simulink model "mapp_4_fir_4_str"  (R2018b)
settings: Solver=ode45  StartTime=0.0  StopTime=200  RelTol=1e-3  EnableMultiTasking=on
undefined symbols (not defined in the file or in its folder): CMD_ci_Re_0, CMD_ci_Re_21, CMD_ci_str_0, CMD_ci_str_1, CMD_ci_str_10, CMD_ci_str_11, CMD_ci_str_12, CMD_ci_str_13, CMD_ci_str_14, CMD_ci_str_15, CMD_ci_str_16, CMD_ci_str_17, CMD_ci_str_18, CMD_ci_str_19, CMD_ci_str_2, CMD_ci_str_20, CMD_ci_str_21, CMD_ci_str_3, CMD_ci_str_4, CMD_ci_str_5, CMD_ci_str_6, CMD_ci_str_7, CMD_ci_str_8, CMD_ci_str_9, CMD_decr_0, CMD_deka_down, CMD_deka_up, CMD_fb, CMD_FB_mult, CMD_Firprg_0, CMD_Firprg_1, CMD_gain, CMD_ind_mult, CMD_ind_mult_1, CMD_ind_mult_2, CMD_ind_mult_3, CMD_ind_mult_4, CMD_ind_stuk, CMD_ind_vol, CMD_ind_vol_1, CMD_ind_vol_2, CMD_ind_vol_3, CMD_ind_vol_4, CMD_init_dac, CMD_init_sw, CMD_molot_string, CMD_nl, CMD_nl_sl, CMD_omega_0, CMD_out_vol, CMD_param_0, CMD_param_5, CMD_pedal, CMD_reset, CMD_rst, CMD_shape_0, CMD_step_down, CMD_step_up, CMD_str_svertk, ind_mult_0 ... (+10)
libraries: xbsIndex_r4 x3300
(part 3 of 16)

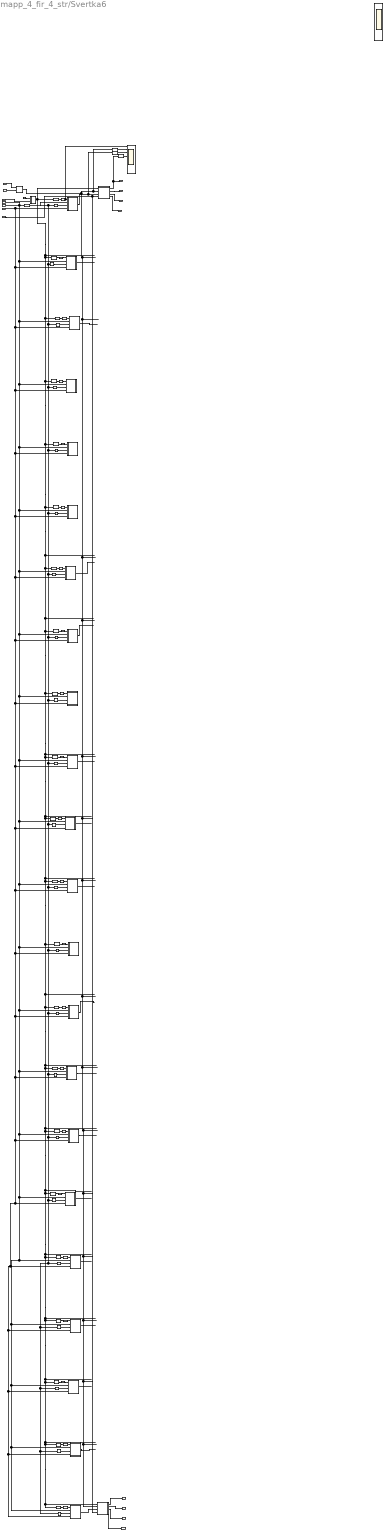
== system mapp_4_fir_4_str/Svertka6 ==
  A_sunn[j] : Inport
  m_dat : Inport  Port=2
  m_addr : Inport  Port=3
  m_en : Inport  Port=4
  start : Inport  Port=5
  FB : Inport  Port=6
  reset : Inport  Port=7
  Constant17 : xbsIndex_r4/Constant  const=531  gui_display_data_type=Fixed-point  arith_type=Unsigned  n_bits=12  bin_pt=0  preci_type=Single  exp_width=8  frac_width=24  explicit_period=off  period=1  equ=P=C  opselect=C  inp2=PCIN>>17  opr=+  inp1=P  carry=CIN  dbl_ovrd=off  block_type=constant
      settings: block_version=VER_STRING_GOES_HERE
  Convert1 : xbsIndex_r4/Convert  gui_display_data_type=Floating-point  arith_type=Floating-point  n_bits=48  bin_pt=0  float_type=Single  exp_bits=8  fraction_bits=24  quantization="Round  (unbiased: +/- Inf)"  overflow=Saturate  en=off  latency=0  pipeline=off  dbl_ovrd=off  block_type=convert
  Convert12 : xbsIndex_r4/Convert  gui_display_data_type=Floating-point  arith_type=Floating-point  n_bits=48  bin_pt=0  float_type=Single  exp_bits=8  fraction_bits=24  quantization="Round  (unbiased: +/- Inf)"  overflow=Saturate  en=off  latency=0  pipeline=off  dbl_ovrd=off  block_type=convert
  Convert2 : xbsIndex_r4/Convert  gui_display_data_type=Floating-point  arith_type=Floating-point  n_bits=48  bin_pt=0  float_type=Single  exp_bits=8  fraction_bits=24  quantization="Round  (unbiased: +/- Inf)"  overflow=Saturate  en=off  latency=0  pipeline=off  dbl_ovrd=off  block_type=convert
  Count : Subsystem
  Delay{1..9,12..16,18..24,278} (22 alike) : xbsIndex_r4/Delay  rst=off  infoeditControl=Selection of Reset will increase slice count due to use of real FFs and instead of SRLs  en=off  latency=127  reg_retiming=off  dbl_ovrd=off  block_type=delay
  Delay{10..11,28,44,58,72,85,100,114,128,141,155,169,182,197,211,225,238,253,267,295,308} (22 alike) : xbsIndex_r4/Delay  rst=off  infoeditControl=Selection of Reset will increase slice count due to use of real FFs and instead of SRLs  en=off  latency=1  reg_retiming=on  dbl_ovrd=off  block_type=delay
      settings: xl_area=[16 32 0 0 0 0 0]  block_version=VER_STRING_GOES_HERE
  Delay{17,27,33,49,63,77,90,105,119,133,146,160,174,187,202,216,230,243,258,272,300,313} (22 alike) : xbsIndex_r4/Delay  rst=off  infoeditControl=Selection of Reset will increase slice count due to use of real FFs and instead of SRLs  en=off  latency=1  reg_retiming=off  dbl_ovrd=off  block_type=delay
  Mult22 : xbsIndex_r4/Mult  precision=Full  arith_type="Signed  (2's comp)"  n_bits=16  bin_pt=14  quantization=Truncate  overflow=Wrap  en=off  latency=6  use_behavioral_HDL=on  opt=Speed  use_embedded=on  optimum_pipeline=off  pipeline=on  dbl_ovrd=off  use_rpm=on  placement_style=Triangular  block_type=mult
  RSlice1 : xbsIndex_r4/Slice  nbits=10  boolean_output=off  mode=Lower Bit Location + Width  bit1=0  base1=MSB of Input  bit0=0  base0=LSB of Input  dbl_ovrd=off  block_type=slice
      settings: block_version=VER_STRING_GOES_HERE
  Scope1 : Scope  NumInputPorts=8
  Scope3 : Scope  NumInputPorts=9
  accum_0 : Subsystem
  accum_1 : Subsystem
  ci_re_0 : Subsystem
  ci_re_1 : Subsystem
  ci_re_10 : Subsystem
  ci_re_11 : Subsystem
  ci_re_12 : Subsystem
  ci_re_13 : Subsystem
  ci_re_14 : Subsystem
  ci_re_15 : Subsystem
  ci_re_16 : Subsystem
  ci_re_17 : Subsystem
  ci_re_18 : Subsystem
  ci_re_19 : Subsystem
  ci_re_2 : Subsystem
  ci_re_20 : Subsystem
  ci_re_21 : Subsystem
  ci_re_3 : Subsystem
  ci_re_4 : Subsystem
  ci_re_5 : Subsystem
  ci_re_6 : Subsystem
  ci_re_7 : Subsystem
  ci_re_8 : Subsystem
  ci_re_9 : Subsystem
  nota_0 : Outport
  nota_87 : Outport  Port=2
  nota_1 : Outport  Port=3
  nota_86 : Outport  Port=4
  nota_2 : Outport  Port=5
  nota_85 : Outport  Port=6
  nota_3 : Outport  Port=7
  nota_84 : Outport  Port=8
  wires:
  start/1 -> Count/2(start)
  Delay27/1 -> Scope3/1, ci_re_0/1(addr)
  m_en/1 -> ci_re_0/4(m_en), ci_re_1/4(m_en), ci_re_6/4(m_en), ci_re_7/4(m_en), ci_re_9/4(m_en), ci_re_10/4(m_en), ci_re_11/4(m_en), ci_re_12/4(m_en), ci_re_13/4(m_en), ci_re_14/4(m_en), ci_re_15/4(m_en), ci_re_16/4(m_en), ci_re_18/4(m_en), ci_re_19/4(m_en), ci_re_20/4(m_en), ci_re_21/4(m_en), ci_re_17/4(m_en), ci_re_8/4(m_en), ci_re_5/4(m_en), ci_re_4/4(m_en), ci_re_3/4(m_en), ci_re_2/4(m_en)
  Delay7/1 -> Delay27/1
  Constant17/1 -> Count/1(In1)
  m_addr/1 -> RSlice1/1
  Delay24/1 -> Delay17/1
  Delay17/1 -> ci_re_1/1(addr)
  Delay33/1 -> ci_re_2/1(addr)
  Delay23/1 -> Delay33/1
  Delay28/1 -> ci_re_2/3(m_addr)
  Delay44/1 -> ci_re_3/3(m_addr)
  Delay22/1 -> Delay49/1
  Delay49/1 -> ci_re_3/1(addr)
  Delay63/1 -> ci_re_4/1(addr)
  Delay21/1 -> Delay63/1
  Delay58/1 -> ci_re_4/3(m_addr)
  Delay77/1 -> ci_re_5/1(addr)
  Delay20/1 -> Delay77/1
  Delay72/1 -> ci_re_5/3(m_addr)
  Delay128/1 -> ci_re_9/3(m_addr)
  Delay15/1 -> Delay133/1
  Delay133/1 -> ci_re_9/1(addr)
  Delay114/1 -> ci_re_8/3(m_addr)
  Delay16/1 -> Delay119/1
  Delay119/1 -> ci_re_8/1(addr)
  Delay105/1 -> ci_re_7/1(addr)
  Delay18/1 -> Delay105/1
  Delay100/1 -> ci_re_7/3(m_addr)
  Delay85/1 -> ci_re_6/3(m_addr)
  Delay19/1 -> Delay90/1
  Delay90/1 -> ci_re_6/1(addr)
  Delay243/1 -> ci_re_14/1(addr)
  Delay238/1 -> ci_re_14/3(m_addr)
  Delay141/1 -> ci_re_15/3(m_addr)
  Delay146/1 -> ci_re_15/1(addr)
  Delay6/1 -> Delay146/1
  Delay160/1 -> ci_re_16/1(addr)
  Delay155/1 -> ci_re_16/3(m_addr)
  Delay5/1 -> Delay160/1
  Delay211/1 -> ci_re_12/3(m_addr)
  Delay216/1 -> ci_re_12/1(addr)
  Delay12/1 -> Delay216/1
  Delay174/1 -> ci_re_17/1(addr)
  Delay169/1 -> ci_re_17/3(m_addr)
  Delay4/1 -> Delay174/1
  Delay202/1 -> ci_re_11/1(addr)
  Delay13/1 -> Delay202/1
  Delay197/1 -> ci_re_11/3(m_addr)
  Delay8/1 -> Delay243/1
  Delay14/1 -> Delay187/1
  Delay187/1 -> ci_re_10/1(addr)
  Delay182/1 -> ci_re_10/3(m_addr)
  Delay230/1 -> ci_re_13/1(addr)
  Delay9/1 -> Delay230/1
  Delay225/1 -> ci_re_13/3(m_addr)
  Delay278/1 -> Delay272/1
  Delay272/1 -> ci_re_21/1(addr)
  RSlice1/1 -> Delay10/1, Delay11/1, Delay28/1, Delay44/1, Delay58/1, Delay72/1, Delay85/1, Delay100/1, Delay114/1, Delay128/1, Delay182/1, Delay238/1, Delay141/1, Delay155/1, Delay295/1, Delay308/1, Delay253/1, Delay267/1, Delay169/1, Delay225/1, Delay211/1, Delay197/1
  Delay258/1 -> ci_re_20/1(addr)
  Delay253/1 -> ci_re_20/3(m_addr)
  Delay313/1 -> ci_re_19/1(addr)
  Delay1/1 -> Delay258/1
  Delay295/1 -> ci_re_18/3(m_addr)
  Delay3/1 -> Delay300/1
  Delay300/1 -> ci_re_18/1(addr)
  Count/1(Out1) -> Delay24/1, Delay23/1, Delay22/1, Delay21/1, Delay20/1, Delay19/1, Delay18/1, Delay16/1, Delay15/1, Delay14/1, Delay13/1, Delay12/1, Delay9/1, Delay8/1, Delay6/1, Delay5/1, Delay4/1, Delay3/1, Delay2/1, Delay1/1, Delay278/1, accum_1/1(In1), accum_0/1(In1), Delay7/1
  Delay308/1 -> ci_re_19/3(m_addr)
  Delay2/1 -> Delay313/1
  m_dat/1 -> ci_re_1/2(m_data), ci_re_2/2(m_data), ci_re_3/2(m_data), ci_re_4/2(m_data), ci_re_5/2(m_data), ci_re_6/2(m_data), ci_re_7/2(m_data), ci_re_8/2(m_data), ci_re_9/2(m_data), ci_re_10/2(m_data), ci_re_11/2(m_data), ci_re_12/2(m_data), ci_re_14/2(m_data), ci_re_15/2(m_data), ci_re_16/2(m_data), ci_re_19/2(m_data), ci_re_20/2(m_data), ci_re_21/2(m_data), ci_re_18/2(m_data), ci_re_17/2(m_data), ci_re_13/2(m_data), ci_re_0/2(m_data)
  Delay10/1 -> ci_re_0/3(m_addr)
  Delay11/1 -> ci_re_1/3(m_addr)
  Delay267/1 -> ci_re_21/3(m_addr)
  Mult22/1 -> Convert12/1, accum_0/2(sig), accum_1/2(sig)
  A_sunn[j]/1 -> Mult22/2
  FB/1 -> Mult22/1
  ci_re_2/1(Out) -> ?
  ci_re_1/1(Out) -> ?
  ci_re_0/1(Out) -> Convert1/1, accum_0/3(coeff)
  accum_0/2(Out2) -> nota_1/1
  accum_0/3(Out3) -> nota_2/1
  accum_0/1(Out1) -> Convert2/1, nota_0/1
  accum_0/4(Out4) -> nota_3/1
  ci_re_6/1(Out) -> ?
  ci_re_7/1(Out) -> ?
  ci_re_9/1(Out) -> ?
  ci_re_11/1(Out) -> ?
  ci_re_10/1(Out) -> ?
  ci_re_13/1(Out) -> ?
  ci_re_14/1(Out) -> ?
  ci_re_15/1(Out) -> ?
  ci_re_16/1(Out) -> ?
  ci_re_17/1(Out) -> ?
  ci_re_18/1(Out) -> ?
  ci_re_19/1(Out) -> ?
  ci_re_20/1(Out) -> ?
  ci_re_21/1(Out) -> accum_1/3(coeff)
  accum_1/2(Out2) -> nota_85/1
  accum_1/1(Out1) -> nota_84/1
  accum_1/3(Out3) -> nota_86/1
  accum_1/4(Out4) -> nota_87/1
  reset/1 -> accum_1/4(reset), accum_0/4(reset)
  Convert12/1 -> Scope3/2
  Convert1/1 -> Scope3/3
  Convert2/1 -> Scope3/4

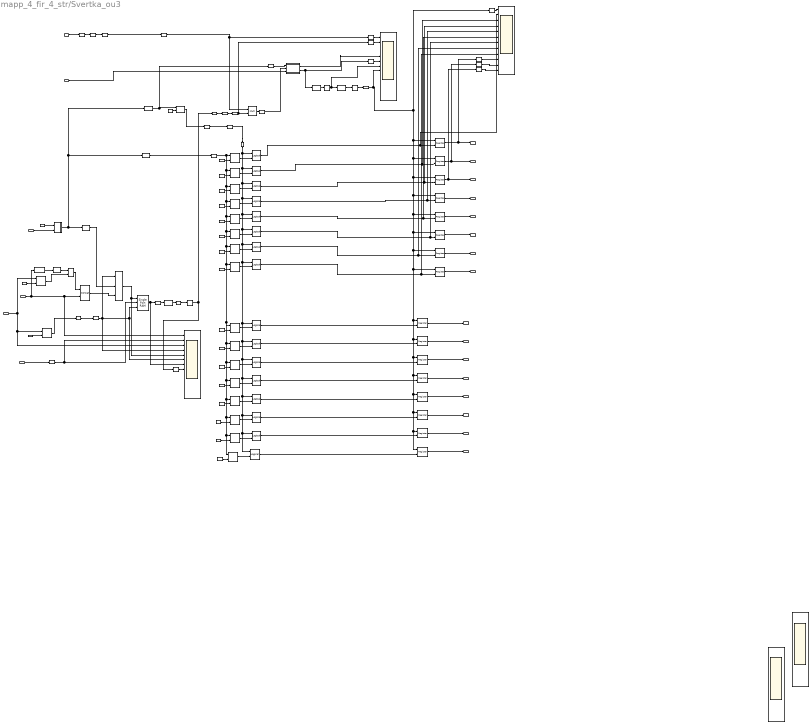
== system mapp_4_fir_4_str/Svertka_ou3 ==
  Osc_summ1 : Inport
  m_dat : Inport  Port=2
  m_addr : Inport  Port=3
  m_en : Inport  Port=4
  start : Inport  Port=5
  reset : Inport  Port=6
  Accum_fl : Subsystem
  CMD_deka_down : xbsIndex_r4/Constant  const=CMD_deka_down  gui_display_data_type=Fixed-point  arith_type=Unsigned  n_bits=8  bin_pt=0  preci_type=Single  exp_width=8  frac_width=24  explicit_period=on  period=1  equ=P=C  opselect=C  inp2=PCIN>>17  opr=+  inp1=P  carry=CIN  dbl_ovrd=off  block_type=constant
      settings: block_version=VER_STRING_GOES_HERE
  CMD_deka_up : xbsIndex_r4/Constant  const=CMD_deka_up  gui_display_data_type=Fixed-point  arith_type=Unsigned  n_bits=8  bin_pt=0  preci_type=Single  exp_width=8  frac_width=24  explicit_period=on  period=1  equ=P=C  opselect=C  inp2=PCIN>>17  opr=+  inp1=P  carry=CIN  dbl_ovrd=off  block_type=constant
      settings: block_version=VER_STRING_GOES_HERE
  Concat : xbsIndex_r4/Concat  num_inputs=2  dbl_ovrd=off  block_type=concat
  Constant1 : xbsIndex_r4/Constant  const=1  gui_display_data_type=Fixed-point  arith_type=Unsigned  n_bits=4  bin_pt=0  preci_type=Single  exp_width=8  frac_width=24  explicit_period=on  period=1  equ=P=C  opselect=C  inp2=PCIN>>17  opr=+  inp1=P  carry=CIN  dbl_ovrd=off  block_type=constant
      settings: block_version=VER_STRING_GOES_HERE
  Constant17 : xbsIndex_r4/Constant  const=400 - 80 - 256  gui_display_data_type=Fixed-point  arith_type=Unsigned  n_bits=12  bin_pt=0  preci_type=Single  exp_width=8  frac_width=24  explicit_period=off  period=1  equ=P=C  opselect=C  inp2=PCIN>>17  opr=+  inp1=P  carry=CIN  dbl_ovrd=off  block_type=constant
      settings: block_version=VER_STRING_GOES_HERE
  Constant2 : xbsIndex_r4/Constant  const=2  gui_display_data_type=Fixed-point  arith_type=Unsigned  n_bits=4  bin_pt=0  preci_type=Single  exp_width=8  frac_width=24  explicit_period=on  period=1  equ=P=C  opselect=C  inp2=PCIN>>17  opr=+  inp1=P  carry=CIN  dbl_ovrd=off  block_type=constant
      settings: block_version=VER_STRING_GOES_HERE
  Constant20 : xbsIndex_r4/Constant  const=6  gui_display_data_type=Fixed-point  arith_type=Signed (2's comp)  n_bits=8  bin_pt=0  preci_type=Single  exp_width=8  frac_width=24  explicit_period=on  period=1  equ=P=C  opselect=C  inp2=PCIN>>17  opr=+  inp1=P  carry=CIN  dbl_ovrd=off  block_type=constant
      settings: block_version=VER_STRING_GOES_HERE
  Constant22 : xbsIndex_r4/Constant  const=1  gui_display_data_type=Fixed-point  arith_type=Unsigned  n_bits=4  bin_pt=0  preci_type=Single  exp_width=8  frac_width=24  explicit_period=on  period=1  equ=P=C  opselect=C  inp2=PCIN>>17  opr=+  inp1=P  carry=CIN  dbl_ovrd=off  block_type=constant
      settings: block_version=VER_STRING_GOES_HERE
  Constant23 : xbsIndex_r4/Constant  const=2  gui_display_data_type=Fixed-point  arith_type=Unsigned  n_bits=4  bin_pt=0  preci_type=Single  exp_width=8  frac_width=24  explicit_period=on  period=1  equ=P=C  opselect=C  inp2=PCIN>>17  opr=+  inp1=P  carry=CIN  dbl_ovrd=off  block_type=constant
      settings: block_version=VER_STRING_GOES_HERE
  Constant24 : xbsIndex_r4/Constant  const=3  gui_display_data_type=Fixed-point  arith_type=Unsigned  n_bits=4  bin_pt=0  preci_type=Single  exp_width=8  frac_width=24  explicit_period=on  period=1  equ=P=C  opselect=C  inp2=PCIN>>17  opr=+  inp1=P  carry=CIN  dbl_ovrd=off  block_type=constant
      settings: block_version=VER_STRING_GOES_HERE
  Constant25 : xbsIndex_r4/Constant  const=4  gui_display_data_type=Fixed-point  arith_type=Unsigned  n_bits=4  bin_pt=0  preci_type=Single  exp_width=8  frac_width=24  explicit_period=on  period=1  equ=P=C  opselect=C  inp2=PCIN>>17  opr=+  inp1=P  carry=CIN  dbl_ovrd=off  block_type=constant
      settings: block_version=VER_STRING_GOES_HERE
  Constant26 : xbsIndex_r4/Constant  const=5  gui_display_data_type=Fixed-point  arith_type=Unsigned  n_bits=4  bin_pt=0  preci_type=Single  exp_width=8  frac_width=24  explicit_period=on  period=1  equ=P=C  opselect=C  inp2=PCIN>>17  opr=+  inp1=P  carry=CIN  dbl_ovrd=off  block_type=constant
      settings: block_version=VER_STRING_GOES_HERE
  Constant27 : xbsIndex_r4/Constant  const=6  gui_display_data_type=Fixed-point  arith_type=Unsigned  n_bits=4  bin_pt=0  preci_type=Single  exp_width=8  frac_width=24  explicit_period=on  period=1  equ=P=C  opselect=C  inp2=PCIN>>17  opr=+  inp1=P  carry=CIN  dbl_ovrd=off  block_type=constant
      settings: block_version=VER_STRING_GOES_HERE
  Constant28 : xbsIndex_r4/Constant  const=7  gui_display_data_type=Fixed-point  arith_type=Unsigned  n_bits=4  bin_pt=0  preci_type=Single  exp_width=8  frac_width=24  explicit_period=on  period=1  equ=P=C  opselect=C  inp2=PCIN>>17  opr=+  inp1=P  carry=CIN  dbl_ovrd=off  block_type=constant
      settings: block_version=VER_STRING_GOES_HERE
  Constant29 : xbsIndex_r4/Constant  const=0  gui_display_data_type=Fixed-point  arith_type=Unsigned  n_bits=4  bin_pt=0  preci_type=Single  exp_width=8  frac_width=24  explicit_period=on  period=1  equ=P=C  opselect=C  inp2=PCIN>>17  opr=+  inp1=P  carry=CIN  dbl_ovrd=off  block_type=constant
      settings: block_version=VER_STRING_GOES_HERE
  Constant3 : xbsIndex_r4/Constant  const=3  gui_display_data_type=Fixed-point  arith_type=Unsigned  n_bits=4  bin_pt=0  preci_type=Single  exp_width=8  frac_width=24  explicit_period=on  period=1  equ=P=C  opselect=C  inp2=PCIN>>17  opr=+  inp1=P  carry=CIN  dbl_ovrd=off  block_type=constant
      settings: block_version=VER_STRING_GOES_HERE
  Constant4 : xbsIndex_r4/Constant  const=4  gui_display_data_type=Fixed-point  arith_type=Unsigned  n_bits=4  bin_pt=0  preci_type=Single  exp_width=8  frac_width=24  explicit_period=on  period=1  equ=P=C  opselect=C  inp2=PCIN>>17  opr=+  inp1=P  carry=CIN  dbl_ovrd=off  block_type=constant
      settings: block_version=VER_STRING_GOES_HERE
  Constant5 : xbsIndex_r4/Constant  const=5  gui_display_data_type=Fixed-point  arith_type=Unsigned  n_bits=4  bin_pt=0  preci_type=Single  exp_width=8  frac_width=24  explicit_period=on  period=1  equ=P=C  opselect=C  inp2=PCIN>>17  opr=+  inp1=P  carry=CIN  dbl_ovrd=off  block_type=constant
      settings: block_version=VER_STRING_GOES_HERE
  Constant6 : xbsIndex_r4/Constant  const=6  gui_display_data_type=Fixed-point  arith_type=Unsigned  n_bits=4  bin_pt=0  preci_type=Single  exp_width=8  frac_width=24  explicit_period=on  period=1  equ=P=C  opselect=C  inp2=PCIN>>17  opr=+  inp1=P  carry=CIN  dbl_ovrd=off  block_type=constant
      settings: block_version=VER_STRING_GOES_HERE
  Constant7 : xbsIndex_r4/Constant  const=7  gui_display_data_type=Fixed-point  arith_type=Unsigned  n_bits=4  bin_pt=0  preci_type=Single  exp_width=8  frac_width=24  explicit_period=on  period=1  equ=P=C  opselect=C  inp2=PCIN>>17  opr=+  inp1=P  carry=CIN  dbl_ovrd=off  block_type=constant
      settings: block_version=VER_STRING_GOES_HERE
  Constant8 : xbsIndex_r4/Constant  const=0  gui_display_data_type=Fixed-point  arith_type=Unsigned  n_bits=4  bin_pt=0  preci_type=Single  exp_width=8  frac_width=24  explicit_period=on  period=1  equ=P=C  opselect=C  inp2=PCIN>>17  opr=+  inp1=P  carry=CIN  dbl_ovrd=off  block_type=constant
      settings: block_version=VER_STRING_GOES_HERE
  Convert : xbsIndex_r4/Convert  gui_display_data_type=Fixed-point  arith_type=Unsigned  n_bits=1  bin_pt=0  float_type=Single  exp_bits=8  fraction_bits=24  quantization=Truncate  overflow=Wrap  en=off  latency=0  pipeline=off  dbl_ovrd=off  block_type=convert
  Convert1 : xbsIndex_r4/Convert  gui_display_data_type=Floating-point  arith_type=Floating-point  n_bits=16  bin_pt=14  float_type=Single  exp_bits=8  fraction_bits=24  quantization=Truncate  overflow=Wrap  en=off  latency=6  pipeline=off  dbl_ovrd=off  block_type=convert
  Convert{2,4,6..11} (8 alike) : xbsIndex_r4/Convert  gui_display_data_type=Floating-point  arith_type=Floating-point  n_bits=16  bin_pt=14  float_type=Single  exp_bits=8  fraction_bits=24  quantization=Truncate  overflow=Wrap  en=off  latency=0  pipeline=off  dbl_ovrd=off  block_type=convert
  Convert12 : xbsIndex_r4/Convert  gui_display_data_type=Fixed-point  arith_type="Signed  (2's comp)"  n_bits=48  bin_pt=24  float_type=Single  exp_bits=8  fraction_bits=24  quantization="Round  (unbiased: +/- Inf)"  overflow=Saturate  en=off  latency=6  pipeline=off  dbl_ovrd=off  block_type=convert
  Count : Subsystem
  Delay{1..6,8,10,12,15,18..19,25} (13 alike) : xbsIndex_r4/Delay  rst=off  infoeditControl=Selection of Reset will increase slice count due to use of real FFs and instead of SRLs  en=off  latency=1  reg_retiming=off  dbl_ovrd=off  block_type=delay
  Delay11 : xbsIndex_r4/Delay  rst=off  infoeditControl=Selection of Reset will increase slice count due to use of real FFs and instead of SRLs  en=off  latency=6  reg_retiming=off  dbl_ovrd=off  block_type=delay
  Delay14 : xbsIndex_r4/Delay  rst=off  infoeditControl=Selection of Reset will increase slice count due to use of real FFs and instead of SRLs  en=off  latency=6  reg_retiming=off  dbl_ovrd=off  block_type=delay
  Delay16 : xbsIndex_r4/Delay  rst=off  infoeditControl=Selection of Reset will increase slice count due to use of real FFs and instead of SRLs  en=off  latency=5  reg_retiming=off  dbl_ovrd=off  block_type=delay
  Delay17 : xbsIndex_r4/Delay  rst=off  infoeditControl=Selection of Reset will increase slice count due to use of real FFs and instead of SRLs  en=off  latency=17  reg_retiming=off  dbl_ovrd=off  block_type=delay
  Delay21 : xbsIndex_r4/Delay  rst=off  infoeditControl=Selection of Reset will increase slice count due to use of real FFs and instead of SRLs  en=off  latency=14  reg_retiming=off  dbl_ovrd=off  block_type=delay
  Logical{2..17} (16 alike) : xbsIndex_r4/Logical  logical_function=AND  inputs=2  en=off  latency=1  precision=Full  arith_type=Unsigned  n_bits=16  bin_pt=0  align_bp=on  dbl_ovrd=off  block_type=logical
  Mult1 : xbsIndex_r4/Mult  precision=Full  arith_type="Signed  (2's comp)"  n_bits=16  bin_pt=14  quantization=Truncate  overflow=Wrap  en=off  latency=6  use_behavioral_HDL=off  opt=Speed  use_embedded=on  optimum_pipeline=off  pipeline=on  dbl_ovrd=off  use_rpm=on  placement_style=Triangular  block_type=mult
  Mux3 : xbsIndex_r4/Mux  inputs=2  en=off  latency=0  precision=Full  arith_type=Unsigned  n_bits=16  bin_pt=14  quantization=Truncate  overflow=Wrap  dbl_ovrd=off  block_type=mux
  RSlice2 : xbsIndex_r4/Slice  nbits=11  boolean_output=off  mode=Lower Bit Location + Width  bit1=0  base1=MSB of Input  bit0=0  base0=LSB of Input  dbl_ovrd=off  block_type=slice
      settings: block_version=VER_STRING_GOES_HERE
  RSlice5 : xbsIndex_r4/Slice  nbits=3  boolean_output=off  mode=Lower Bit Location + Width  bit1=0  base1=MSB of Input  bit0=8  base0=LSB of Input  dbl_ovrd=off  block_type=slice
      settings: block_version=VER_STRING_GOES_HERE
  RSlice6 : xbsIndex_r4/Slice  nbits=8  boolean_output=off  mode=Lower Bit Location + Width  bit1=0  base1=MSB of Input  bit0=0  base0=LSB of Input  dbl_ovrd=off  block_type=slice
      settings: block_version=VER_STRING_GOES_HERE
  Register{,3..4,6..19} (17 alike) : xbsIndex_r4/Register  init=0  rst=off  en=on  dbl_ovrd=off  block_type=register
  Register2 : xbsIndex_r4/Register  init=0  rst=off  en=off  dbl_ovrd=off  block_type=register
  Reinterpret : xbsIndex_r4/Reinterpret  force_arith_type=on  arith_type=Floating-point  force_bin_pt=on  bin_pt=24  block_type=reinterpret
  Reinterpret3 : xbsIndex_r4/Reinterpret  force_arith_type=on  arith_type="Signed  (2's comp)"  force_bin_pt=on  bin_pt=0  block_type=reinterpret
  Reinterpret4 : xbsIndex_r4/Reinterpret  force_arith_type=on  arith_type="Signed  (2's comp)"  force_bin_pt=on  bin_pt=0  block_type=reinterpret
  Relational{,10..25} (17 alike) : xbsIndex_r4/Relational  mode=a=b  op_type=Bool  en=off  latency=1  dbl_ovrd=off  block_type=relational
      Relational10 settings: xl_area=[4 1 0 7 0 0 0]  block_version=VER_STRING_GOES_HERE
  Relational1 : xbsIndex_r4/Relational  mode=a=b  op_type=Bool  en=off  latency=0  dbl_ovrd=off  block_type=relational
  Relational2 : xbsIndex_r4/Relational  mode=a=b  op_type=Bool  en=off  latency=0  dbl_ovrd=off  block_type=relational
  Scope1 : Scope  NumInputPorts=13
  Scope3 : Scope  NumInputPorts=18
  Scope5 : Scope  NumInputPorts=18
  Scope6 : Scope  NumInputPorts=13
  Scope7 : Scope  NumInputPorts=12
  Single Port RAM2 : xbsIndex_r4/Single Port RAM  depth=256*8  initVector=Res2  distributed_mem=Block RAM  write_mode=Read After Write  rst=off  init_reg=0  en=off  latency=1  optimize=Area  dbl_ovrd=off  block_type=spram
  Slice : xbsIndex_r4/Slice  nbits=1  boolean_output=off  mode=Lower Bit Location + Width  bit1=0  base1=MSB of Input  bit0=0  base0=LSB of Input  dbl_ovrd=off  block_type=slice
  Slice1 : xbsIndex_r4/Slice  nbits=24  boolean_output=off  mode=Upper Bit Location + Width  bit1=0  base1=MSB of Input  bit0=8  base0=LSB of Input  dbl_ovrd=off  block_type=slice
  au_0 : Outport
  au_1 : Outport  Port=2
  au_2 : Outport  Port=3
  au_3 : Outport  Port=4
  au_4 : Outport  Port=5
  au_5 : Outport  Port=6
  au_6 : Outport  Port=7
  au_7 : Outport  Port=8
  au_8 : Outport  Port=9
  au_9 : Outport  Port=10
  au_10 : Outport  Port=11
  au_11 : Outport  Port=12
  au_12 : Outport  Port=13
  au_13 : Outport  Port=14
  au_14 : Outport  Port=15
  au_15 : Outport  Port=16
  wires:
  Register8/1 -> au_4/1
  Mult1/1 -> Delay11/1
  Convert/1 -> Register3/1
  Relational17/1 -> Logical9/2
  Register11/1 -> au_7/1
  Register19/1 -> au_8/1
  Register10/1 -> au_6/1
  Logical7/1 -> Scope7/7, Register9/2
  Constant27/1 -> Relational15/2
  Constant25/1 -> Relational13/2
  Constant24/1 -> Relational12/2
  Register7/1 -> au_3/1
  Delay18/1 -> Scope1/8, Register4/1, Register6/1, Register7/1, Register8/1, Register9/1, Register10/1, Register11/1, Register14/1, Register15/1, Register16/1, Register13/1, Register12/1, Register18/1, Register17/1, Register19/1, Register/1, Convert11/1
  Reinterpret4/1 -> Delay18/1
  Constant28/1 -> Relational16/2
  Relational12/1 -> Logical4/2
  Reinterpret/1 -> Delay4/1
  Convert4/1 -> Scope1/2
  Relational10/1 -> Delay21/1
  Relational16/1 -> Logical8/2
  Logical3/1 -> Scope7/3, Register4/2
  Logical4/1 -> Scope7/4, Register6/2
  Constant4/1 -> Relational21/2
  Relational11/1 -> Logical3/2
  Delay4/1 -> Convert1/1
  Logical6/1 -> Scope7/6, Register8/2
  Constant2/1 -> Relational19/2
  Delay12/1 -> Delay2/1
  Delay5/1 -> Delay19/1
  Relational20/1 -> Logical12/2
  Logical5/1 -> Scope7/5, Register7/2
  Relational/1 -> Logical2/2
  Convert8/1 -> Scope7/12
  Constant23/1 -> Relational11/2
  Constant29/1 -> Relational17/2
  Logical14/1 -> Register17/2
  CMD_deka_down/1 -> Relational2/2
  Constant22/1 -> Relational/2
  Delay8/1 -> Delay5/1
  Slice/1 -> Convert/1
  Delay1/1 -> Delay10/1
  Relational19/1 -> Logical11/2
  Count/1(Out1) -> RSlice2/1, RSlice5/1, RSlice6/1
  CMD_deka_up/1 -> Relational1/2
  Osc_summ1/1 -> Register2/1
  Register/1 -> Convert10/1, au_0/1
  Logical17/1 -> Register13/2
  RSlice5/1 -> Delay25/1
  Relational2/1 -> Delay1/1
  RSlice6/1 -> Delay16/1, Relational10/1
  Constant26/1 -> Relational14/2
  Relational1/1 -> Register3/2
  Delay11/1 -> Accum_fl/2(sig)
  Convert9/1 -> Scope7/11
  Register9/1 -> au_5/1
  Register13/1 -> au_15/1
  Relational24/1 -> Logical16/2
  Delay17/1 -> Delay12/1
  Constant6/1 -> Relational23/2
  Relational14/1 -> Logical6/2
  Delay15/1 -> Delay14/1
  Register18/1 -> au_13/1
  Logical8/1 -> Scope7/8, Register10/2
  Register12/1 -> au_14/1
  Logical9/1 -> Scope7/9, Register11/2
  Constant1/1 -> Relational18/2
  Logical11/1 -> Register14/2
  Convert7/1 -> Scope6/8
  Register17/1 -> au_12/1
  Reinterpret3/1 -> Scope1/7, Slice1/1
  Mux3/1 -> Scope6/5, Single Port RAM2/1
  Register16/1 -> au_11/1
  Accum_fl/2(sig_out) -> Convert12/1, Convert6/1
  Relational21/1 -> Logical13/2
  Logical15/1 -> Register18/2
  m_dat/1 -> Delay6/1
  Delay25/1 -> Relational/1, Relational17/1, Relational18/1, Relational19/1, Relational20/1, Relational21/1, Relational22/1, Relational23/1, Relational25/1, Relational24/1, Relational16/1, Relational15/1, Relational14/1, Relational13/1, Relational12/1, Relational11/1
  Register2/1 -> Delay17/1
  Register6/1 -> Convert8/1, au_2/1
  Register14/1 -> au_9/1
  RSlice2/1 -> Mux3/2
  Logical2/1 -> Scope7/2, Register/2
  Register15/1 -> au_10/1
  Convert6/1 -> Scope1/6
  Logical13/1 -> Register16/2
  Convert10/1 -> Scope7/10
  Convert12/1 -> Reinterpret3/1
  Delay14/1 -> Logical2/1, Logical9/1, Logical11/1, Logical12/1, Logical13/1, Logical14/1, Logical15/1, Logical16/1, Logical17/1, Logical10/1, Logical8/1, Logical7/1, Logical6/1, Logical5/1, Logical4/1, Logical3/1
  Delay10/1 -> Scope6/4, Mux3/1, Scope6/6, Single Port RAM2/3
  m_en/1 -> Scope6/3, Relational2/1, Relational1/1
  Delay6/1 -> Scope6/2, Single Port RAM2/2
  Concat/1 -> Mux3/3
  Register4/1 -> Convert9/1, au_1/1
  Register3/1 -> Concat/1
  Relational13/1 -> Logical5/2
  Convert1/1 -> Convert7/1, Delay8/1
  Constant5/1 -> Relational22/2
  Logical12/1 -> Register15/2
  Convert11/1 -> Scope7/1
  Convert2/1 -> Scope1/1
  Slice1/1 -> Reinterpret4/1
  Delay16/1 -> Accum_fl/1(addr_256)
  Delay21/1 -> Delay15/1
  Delay3/1 -> Reinterpret/1
  Single Port RAM2/1 -> Scope6/7, Delay3/1
  start/1 -> Count/2(start)
  Constant20/1 -> Relational10/2
  Relational18/1 -> Logical10/2
  Constant8/1 -> Relational25/2
  Constant7/1 -> Relational24/2
  Delay19/1 -> Convert4/1, Mult1/2
  Constant17/1 -> Count/1(In1)
  Relational22/1 -> Logical14/2
  Constant3/1 -> Relational20/2
  Logical10/1 -> Register19/2
  Accum_fl/1(strb) -> Scope1/5
  m_addr/1 -> Scope6/1, Concat/2, Slice/1
  Relational15/1 -> Logical7/2
  Relational23/1 -> Logical15/2
  Relational25/1 -> Logical17/2
  Logical16/1 -> Register12/2
  Delay2/1 -> Mult1/1, Convert2/1
  reset/1 -> Accum_fl/3(reset)

== system mapp_4_fir_4_str/en1 ==
  In1 : Inport
  Delay : xbsIndex_r4/Delay  rst=off  infoeditControl=Selection of Reset will increase slice count due to use of real FFs and instead of SRLs  en=off  latency=1  reg_retiming=off  dbl_ovrd=off  block_type=delay
  Logical : xbsIndex_r4/Logical  logical_function=AND  inputs=2  en=off  latency=0  precision=Full  arith_type=Unsigned  n_bits=16  bin_pt=0  align_bp=on  dbl_ovrd=off  block_type=logical
  Logical1 : xbsIndex_r4/Logical  logical_function=XOR  inputs=2  en=off  latency=0  precision=Full  arith_type=Unsigned  n_bits=16  bin_pt=0  align_bp=on  dbl_ovrd=off  block_type=logical
  Out1 : Outport
  wires:
  In1/1 -> Logical/1, Delay/1, Logical1/2
  Logical/1 -> Out1/1
  Delay/1 -> Logical1/1
  Logical1/1 -> Logical/2

== system mapp_4_fir_4_str/en2 ==
  In1 : Inport
  Delay : xbsIndex_r4/Delay  rst=off  infoeditControl=Selection of Reset will increase slice count due to use of real FFs and instead of SRLs  en=off  latency=1  reg_retiming=off  dbl_ovrd=off  block_type=delay
  Logical : xbsIndex_r4/Logical  logical_function=AND  inputs=2  en=off  latency=0  precision=Full  arith_type=Unsigned  n_bits=16  bin_pt=0  align_bp=on  dbl_ovrd=off  block_type=logical
  Logical1 : xbsIndex_r4/Logical  logical_function=XOR  inputs=2  en=off  latency=0  precision=Full  arith_type=Unsigned  n_bits=16  bin_pt=0  align_bp=on  dbl_ovrd=off  block_type=logical
  Out1 : Outport
  wires:
  Logical1/1 -> Logical/2
  Delay/1 -> Logical1/1
  Logical/1 -> Out1/1
  In1/1 -> Logical1/2, Delay/1, Logical/1

== system mapp_4_fir_4_str/mashinka_0 ==
  Addr_param : Inport
  Dat_param : Inport  Port=2
  we_param : Inport  Port=3
  Addr : Inport  Port=4
  force : Inport  Port=5
  NN : Inport  Port=6
  Pedal : Inport  Port=7
  Reset : Inport  Port=8
  start : Inport  Port=9
  nn_fl : Inport  Port=10
  LASTX0 : Inport  Port=11
  LASTX1 : Inport  Port=12
  LASTX2 : Inport  Port=13
  LASTX3 : Inport  Port=14
  Constant1 : xbsIndex_r4/Constant  const=0  gui_display_data_type=Floating-point  arith_type=Floating-point  n_bits=16  bin_pt=14  preci_type=Single  exp_width=8  frac_width=24  explicit_period=on  period=1  equ=P=C  opselect=C  inp2=PCIN>>17  opr=+  inp1=P  carry=CIN  dbl_ovrd=off  block_type=constant
  Force_str0 : Subsystem  mask{num_str_12=num_str0, num_point_256=num_pts0, num_param=9, num_harm_32=num_harm_0}
      mask prompts: num_str_12 "num of strings"; num_point_256 "num of points"; num_param "num param"; num_harm_32 "num harms"
  RSlice4 : xbsIndex_r4/Slice  nbits=24  boolean_output=off  mode=Lower Bit Location + Width  bit1=0  base1=MSB of Input  bit0=0  base0=LSB of Input  dbl_ovrd=off  block_type=slice
      settings: block_version=VER_STRING_GOES_HERE
  Register{1,68..75} (9 alike) : xbsIndex_r4/Register  init=0  rst=off  en=off  dbl_ovrd=off  block_type=register
  Reinterpret2 : xbsIndex_r4/Reinterpret  force_arith_type=on  arith_type=Unsigned  force_bin_pt=on  bin_pt=0  block_type=reinterpret
  out_0 : Outport
  out_1 : Outport  Port=2
  out_2 : Outport  Port=3
  out_3 : Outport  Port=4
  wires:
  Force_str0/4(Force_nota3) -> out_3/1
  Force_str0/3(Force_nota2) -> out_2/1
  Force_str0/2(Force_nota1) -> out_1/1
  Force_str0/1(Force_nota0) -> out_0/1
  Register1/1 -> Force_str0/10(nn_fl)
  nn_fl/1 -> Register1/1
  start/1 -> Force_str0/9(start)
  RSlice4/1 -> Reinterpret2/1
  Register71/1 -> Force_str0/7(Pedal)
  Register68/1 -> Force_str0/1(Force_in)
  Register73/1 -> Force_str0/2(NN_in)
  Register70/1 -> Force_str0/8(Reset)
  Register74/1 -> Force_str0/5(Dat_param)
  Register69/1 -> Force_str0/3(Addr)
  Register75/1 -> Force_str0/4(Addr_param)
  Register72/1 -> Force_str0/6(we_param)
  NN/1 -> Register73/1
  Pedal/1 -> Register71/1
  we_param/1 -> Register72/1
  force/1 -> Register68/1
  Reset/1 -> Register70/1
  Addr/1 -> Register69/1
  Dat_param/1 -> RSlice4/1
  Addr_param/1 -> Register75/1
  Reinterpret2/1 -> Register74/1
  LASTX0/1 -> Force_str0/11(LASTX0)
  LASTX3/1 -> Force_str0/14(LASTX3)
  LASTX1/1 -> Force_str0/12(LASTX1)
  LASTX2/1 -> Force_str0/13(LASTX2)
